simulink model "hpt_topology1_tutorial"  (R2025a)
settings: Solver=FixedStepDiscrete  StartTime=0.0  StopTime=0.25  FixedStep=Ts_power  RelTol=1e-3
model workspace (MAT data in the model file):
  Cdc_nom = 0.0022
  I_energy_max = 220
  K_vdc = 0.0018
  K_vreg = -0.03
  L_w5_open = 0
  Lg_grid = 0.262592258879
  P_load = 400000
  Q_load_cap = 0
  Q_load_ind = 0
  R_w4_open = 1000000000
  R_w5_open = 1000000000
  Rg_grid = 11.7851130198
  SCR_grid = 3
  S_base = 400000
  S_energy = 120000
  S_main = 400000
  S_series = 30000
  Ts_power = 2e-05
  Vaux_LL = 400
  Vdc_chopper_on = 850
  Vdc_neg_ref = 0
  Vdc_nom = 800
  Vdc_ref = 875
  Vgrid_LL = 11000
  Vinj_w5_phase_peak = 326.598632371
  Vload_LL = 400
  Vlv_LL = 400
  Vlv_ref_phase = 207
  Vmv_LL = 10000
  Vw5_reg = 400
  Vw6_series = 100
  f_grid = 50
  hpt_energy_auto = 1
  hpt_pwm_fs = 2000
  hpt_vreg_auto = 1
  m_energy_limit = 1.5
  m_energy_manual = 0
  m_reg_limit = 0.6
  m_reg_manual = 0
  omega_grid = 314.159265359
  vdc_lpf_alpha = 0.004
  vreg_lpf_alpha = 0.004
libraries: simulink x9, spsLinearTransformerLib x6, spsUniversalBridgeLib x4, spsGroundLib x3, spsThreePhaseVIMeasurementLib x2, spsSeriesRLCBranchLib x1, spsVoltageMeasurementLib x1, spsControlledCurrentSourceLib x1, spsThreePhaseSourceLib x1, spsThreePhaseSeriesRLCLoadLib x1, spsThreePhaseSeriesRLCBranchLib x1, sps_lib x1
settings Model: Creator=m1391  LastModifiedBy=m1391

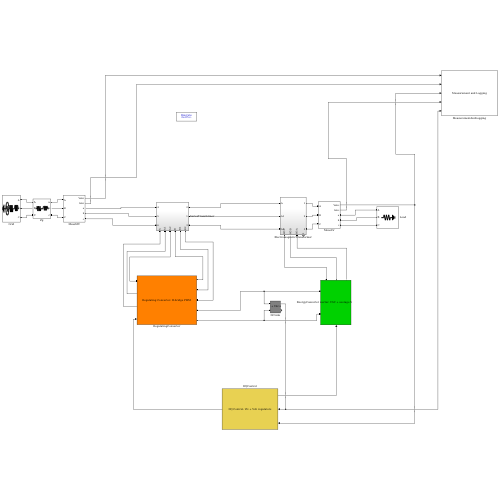
[thumbnail: Simulink's stored preview of the top-level diagram]
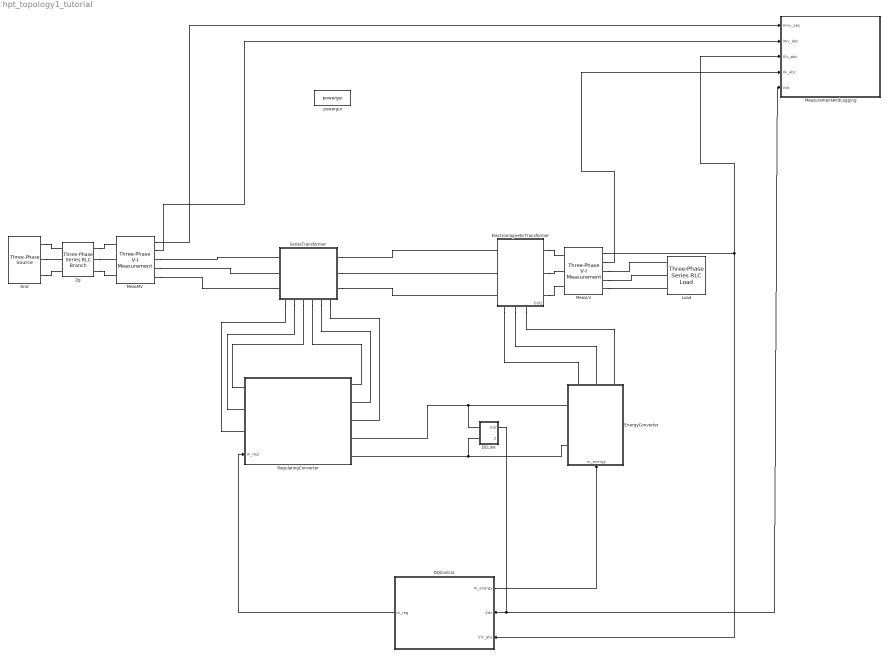
== system hpt_topology1_tutorial ==
  DCLink : Subsystem
      mask Display: disp('DC Link: Cdc + Vdc measurement');
  DQControl : Subsystem
      settings: PortSchema="{\"entries\":[{\"content\":{\"sides\":[{\"content\":{\"connectorIds\":[\"In1\",\"In2\",\"Out2\"]},\"type\":\"ConnectorPlacement.EquallySpacedRectSide\",\"uuid\":\"3cf5f39b-346d-4845-a4cb-051bfc2b4b05\"},{\"content\":{\"connectorIds\":[\"Out1\"],\"side\":\"RIGHT\"},\"type\":\"ConnectorPlacement.EquallySpacedRectSide\",\"uuid\":\"ecd50919-0b1c-4c05-b48e-325f2eadaf48\"},{\"content\":{\"side\":\"TOP\"},\"type\":\"ConnectorPlacement.EquallySpacedRectSide\",\"uuid\":\"d29a4cd4-7c66-4d73-bb68-e387a593270b\"}]},\"type\":\"ConnectorPlacement.EquallySpacedConnector\",\"uuid\":\"966f23e7-eea6-45dc-87ce-60332307e870\"}],\"packageUris\":[\"http://schema.mathworks.com/mf0/Connector/R2020b\"],\"version\":\"1.0\"}"
      mask Display: disp('DQ Control: Vlv + Vdc regulators');
  ElectromagneticTransformer : Subsystem
      settings: PortSchema="{\"entries\":[{\"content\":{\"sides\":[{\"content\":{\"connectorIds\":[\"LConn1\",\"LConn2\",\"LConn3\"]},\"type\":\"ConnectorPlacement.EquallySpacedRectSide\",\"uuid\":\"a1b13bb1-2dce-4e6a-9079-2e847976adb7\"},{\"content\":{\"connectorIds\":[\"RConn1\",\"RConn2\",\"RConn3\"],\"side\":\"RIGHT\"},\"type\":\"ConnectorPlacement.EquallySpacedRectSide\",\"uuid\":\"d74f82ee-ef21-4deb-91b0-5013dd9f5252\"},{\"content\":{\"side\":\"TOP\"},\"type\":\"ConnectorPlacement.EquallySpacedRectSide\",\"uuid\":\"c8027a0e-7a63-44e2-8b0b-a3b1c9bc6e6e\"},{\"content\":{\"connectorIds\":[\"RConn4\",\"RConn5\",\"RConn6\",\"Out1\"],\"side\":\"BOTTOM\"},\"type\":\"ConnectorPlacement.EquallySpacedRectSide\",\"uuid\":\"67c2655b-5962-44e1-8ca2-30aff8808cec\"}]},\"type\":\"ConnectorPlacement.EquallySpacedConnector\",\"uuid\":\"b1661991-e7ef-4d20-9f05-05442b8b5b75\"}],\"packageUris\":[\"http://schema.mathworks.com/mf0/Connector/R2020b\"],\"version\":\"1.0\"}"
  EnergyConverter : Subsystem
      settings: PortSchema="{\"entries\":[{\"content\":{\"sides\":[{\"content\":{\"connectorIds\":[\"LConn1\",\"LConn2\",\"LConn3\"]},\"type\":\"ConnectorPlacement.EquallySpacedRectSide\",\"uuid\":\"97f6e42d-fadd-43ac-9276-7e2aa194abfa\"},{\"content\":{\"connectorIds\":[\"In1\"],\"side\":\"RIGHT\"},\"type\":\"ConnectorPlacement.EquallySpacedRectSide\",\"uuid\":\"de6186ba-5c28-4c9b-a5f0-012c988ed5c8\"},{\"content\":{\"side\":\"TOP\"},\"type\":\"ConnectorPlacement.EquallySpacedRectSide\",\"uuid\":\"44ac97f7-235b-401f-a006-13d9f71848c4\"},{\"content\":{\"connectorIds\":[\"RConn1\",\"RConn2\"],\"side\":\"BOTTOM\"},\"type\":\"ConnectorPlacement.EquallySpacedRectSide\",\"uuid\":\"a31777c4-3c51-48d3-9206-785db4191288\"}]},\"type\":\"ConnectorPlacement.EquallySpacedConnector\",\"uuid\":\"4528e4fd-5330-48b9-923f-21a37255ca08\"}],\"packageUris\":[\"http://schema.mathworks.com/mf0/Connector/R2020b\"],\"version\":\"1.0\"}"
      mask Display: disp('Energy Converter: VSC + average Vdc support');
  Grid : spsThreePhaseSourceLib/Three-Phase Source  InternalConnection=Yg  VoltagePhases=off  Voltage=Vgrid_LL  PhaseAngle=0  Voltage_phases=[25e3 25e3 25e3]/sqrt(3)  PhaseAngles_phases=[0 -120 +120]  Frequency=f_grid  NonIdealSource=on  SpecifyImpedance=off  Resistance=1e-3  Inductance=1e-5  ShortCircuitLevel=100e6  BaseVoltage=25e3  XRratio=7  BusType=swing  Pref=10e3  Qref=0  Prefabc=[10e3, 10e3, 10e3]  Qrefabc=[0, 0, 0]  Qmin=-inf  Qmax=inf
  Load : spsThreePhaseSeriesRLCLoadLib/Three-Phase Series RLC Load  LConnTagsString=A|B|C  Configuration=Y (grounded)  NominalVoltage=Vload_LL  Vabc=[1e3 1e3 1e3]  Vabcp=[1e3 1e3 1e3]  NominalFrequency=f_grid  UnbalancedPower=off  ActivePower=P_load  InductivePower=Q_load_ind  CapacitivePower=Q_load_cap  Pabc=[10e3 9e3 11e3]  QLabc=[100 90 110]  QCabc=[100 90 110]  Pabcp=[10e3 9e3 11e3]  QLabcp=[100 90 110]  QCabcp=[100 90 110]  Measurements=None  LoadType=constant Z
  MeasLV : spsThreePhaseVIMeasurementLib/Three-Phase V-I Measurement  VoltageMeasurement=phase-to-ground  SetLabelV=off  LabelV=Vabc  Vpu=off  VpuLL=off  CurrentMeasurement=yes  SetLabelI=off  LabelI=Iabc  Ipu=off  Pbase=100e6  Vbase=500e3  OutputType=Complex  PhasorSimulation=off  PSBequivalent=0
  MeasMV : spsThreePhaseVIMeasurementLib/Three-Phase V-I Measurement  VoltageMeasurement=phase-to-ground  SetLabelV=off  LabelV=Vabc  Vpu=off  VpuLL=off  CurrentMeasurement=yes  SetLabelI=off  LabelI=Iabc  Ipu=off  Pbase=100e6  Vbase=500e3  OutputType=Complex  PhasorSimulation=off  PSBequivalent=0
  MeasurementAndLogging : Subsystem
      mask Display: disp('Measurement and Logging');
  RegulatingConverter : Subsystem
      settings: PortSchema="{\"entries\":[{\"content\":{\"sides\":[{\"content\":{\"connectorIds\":[\"LConn1\",\"LConn2\",\"LConn3\",\"In1\"]},\"type\":\"ConnectorPlacement.EquallySpacedRectSide\",\"uuid\":\"97f6e42d-fadd-43ac-9276-7e2aa194abfa\"},{\"content\":{\"connectorIds\":[\"RConn1\",\"RConn2\",\"RConn3\",\"RConn4\",\"RConn5\"],\"side\":\"RIGHT\"},\"type\":\"ConnectorPlacement.EquallySpacedRectSide\",\"uuid\":\"de6186ba-5c28-4c9b-a5f0-012c988ed5c8\"},{\"content\":{\"side\":\"TOP\"},\"type\":\"ConnectorPlacement.EquallySpacedRectSide\",\"uuid\":\"44ac97f7-235b-401f-a006-13d9f71848c4\"}]},\"type\":\"ConnectorPlacement.EquallySpacedConnector\",\"uuid\":\"4528e4fd-5330-48b9-923f-21a37255ca08\"}],\"packageUris\":[\"http://schema.mathworks.com/mf0/Connector/R2020b\"],\"version\":\"1.0\"}"
      mask Display: disp('Regulating Converter: H-bridge PWM');
  SeriesTransformer : Subsystem
      settings: PortSchema="{\"entries\":[{\"content\":{\"sides\":[{\"content\":{\"connectorIds\":[\"LConn1\",\"LConn2\",\"LConn3\",\"LConn4\",\"LConn5\",\"LConn6\"]},\"type\":\"ConnectorPlacement.EquallySpacedRectSide\",\"uuid\":\"20d82d84-5695-4c20-a185-fbc9bc49a76c\"},{\"content\":{\"side\":\"RIGHT\"},\"type\":\"ConnectorPlacement.EquallySpacedRectSide\",\"uuid\":\"33b448d8-8c06-4227-825b-ecd8e4ec0e04\"},{\"content\":{\"connectorIds\":[\"LConn7\",\"LConn8\",\"LConn9\"],\"side\":\"TOP\"},\"type\":\"ConnectorPlacement.EquallySpacedRectSide\",\"uuid\":\"ab355161-f222-40c3-9b59-8845a3e0aeb1\"},{\"content\":{\"connectorIds\":[\"RConn1\",\"RConn2\",\"RConn3\"],\"side\":\"BOTTOM\"},\"type\":\"ConnectorPlacement.EquallySpacedRectSide\",\"uuid\":\"91de8b9a-4f62-4b4f-95bb-28c45509e8d0\"}]},\"type\":\"ConnectorPlacement.EquallySpacedConnector\",\"uuid\":\"d2e8fda0-d220-450b-a404-ca6f656a2c35\"}],\"packageUris\":[\"http://schema.mathworks.com/mf0/Connector/R2020b\"],\"version\":\"1.0\"}"
  Zg : spsThreePhaseSeriesRLCBranchLib/Three-Phase Series RLC Branch  LConnTagsString=A|B|C  RConnTagsString=A|B|C  BranchType=RL  Resistance=Rg_grid  Inductance=Lg_grid  Capacitance=1e-6  Measurements=None
  powergui : sps_lib/powergui  Priority=1  SimulationMode=Discrete  SampleTime=Ts_power  frequency=60  Iterations=50  frequencyindice=50  Pbase=100e6  ErrMax=1e-4  UnitsV=kV  UnitsW=MW  buscounter=0  FunctionMessages=off  echomessages=off  EnableUseOfTLC=off  CurrentSourceSwitches=off  DisableSnubberDevices=off  DisableRonSwitches=off  DisableVfSwitches=off  DisplayEquations=off  AutomaticDiscreteSolvers=off  SolverType=Tustin/Backward Euler (TBE)  Interpol=off  ExternalGateDelay=off  methode=off  Ts=100  x0status=blocks  SPID=on  SwTol=0  HookPort=off  NonlinearTolerance=1e-4  nMaxIteration=100  ContinueOnMaxIteration=off  RestoreLinks=warning  ResistiveCurrentMeasurement=off  Frange=[0:2:500]  Ylog=off  Xlog=on  ShowGrid=off  save=off  variable=ZData  structure=0  ZoomFFT=off  StartTime=0.0  cycles=1  DisplayStyle=1  fundamental=60  FreqAxis=off  MaxFrequency=1000  frequencyindicesteady=1  RmsSteady=1  display=off
  wires:
  DCLink/1(Vdc) -> MeasurementAndLogging/5(Vdc), DQControl/2(Vdc)
  MeasMV/1 -> MeasurementAndLogging/1(Vmv_abc)
  MeasMV/2 -> MeasurementAndLogging/2(Imv_abc)
  MeasLV/1 -> MeasurementAndLogging/3(Vlv_abc), DQControl/1(Vlv_abc)
  MeasLV/2 -> MeasurementAndLogging/4(Ilv_abc)
  DQControl/1(m_reg) -> RegulatingConverter/1(m_reg)
  DQControl/2(m_energy) -> EnergyConverter/1(m_energy)
  connections:
  Grid/RConn1 -- Zg/LConn1
  Zg/RConn1 -- MeasMV/LConn1
  Grid/RConn2 -- Zg/LConn2
  Zg/RConn2 -- MeasMV/LConn2
  Grid/RConn3 -- Zg/LConn3
  Zg/RConn3 -- MeasMV/LConn3
  MeasLV/RConn1 -- Load/LConn1
  MeasLV/RConn2 -- Load/LConn2
  MeasLV/RConn3 -- Load/LConn3
  SeriesTransformer/LConn1 -- RegulatingConverter/LConn3
  SeriesTransformer/LConn4 -- RegulatingConverter/RConn1
  SeriesTransformer/LConn2 -- RegulatingConverter/LConn2
  SeriesTransformer/LConn5 -- RegulatingConverter/RConn2
  SeriesTransformer/LConn3 -- RegulatingConverter/LConn1
  SeriesTransformer/LConn6 -- RegulatingConverter/RConn3
  SeriesTransformer/RConn3 -- ElectromagneticTransformer/LConn1
  SeriesTransformer/RConn2 -- ElectromagneticTransformer/LConn2
  SeriesTransformer/RConn1 -- ElectromagneticTransformer/LConn3
  MeasMV/RConn1 -- SeriesTransformer/LConn9
  MeasMV/RConn2 -- SeriesTransformer/LConn8
  MeasMV/RConn3 -- SeriesTransformer/LConn7
  DCLink/LConn1 -- RegulatingConverter/RConn4 -- EnergyConverter/RConn1
  DCLink/LConn2 -- RegulatingConverter/RConn5 -- EnergyConverter/RConn2
  ElectromagneticTransformer/RConn1 -- MeasLV/LConn1
  ElectromagneticTransformer/RConn6 -- EnergyConverter/LConn1
  ElectromagneticTransformer/RConn2 -- MeasLV/LConn2
  ElectromagneticTransformer/RConn5 -- EnergyConverter/LConn2
  ElectromagneticTransformer/RConn3 -- MeasLV/LConn3
  ElectromagneticTransformer/RConn4 -- EnergyConverter/LConn3

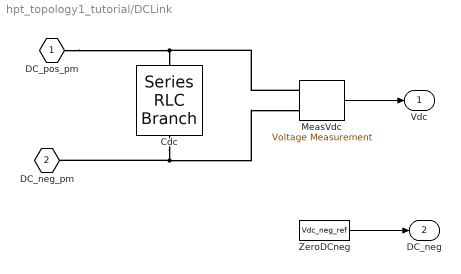
== system hpt_topology1_tutorial/DCLink ==
  Cdc : spsSeriesRLCBranchLib/Series RLC Branch  LConnTagsString=__new0  RConnTagsString=__new0  BranchType=C  Resistance=1  Inductance=1e-3  SetiL0=off  InitialCurrent=0  Capacitance=Cdc_nom  Setx0=off  InitialVoltage=Vdc_nom  Measurements=None
  MeasVdc : spsVoltageMeasurementLib/Voltage Measurement  PhasorSimulation=off  OutputType=Complex  PSBequivalent=0
  ZeroDCneg : Constant  Value=Vdc_neg_ref
  DC_pos_pm : PMIOPort  Side=Left
  DC_neg_pm : PMIOPort  Port=2  Side=Left
  Vdc : Outport
  DC_neg : Outport  Port=2
  wires:
  MeasVdc/1 -> Vdc/1
  ZeroDCneg/1 -> DC_neg/1
  connections:
  DC_pos_pm/RConn1 -- MeasVdc/LConn1 -- Cdc/LConn1
  DC_neg_pm/RConn1 -- MeasVdc/LConn2 -- Cdc/RConn1

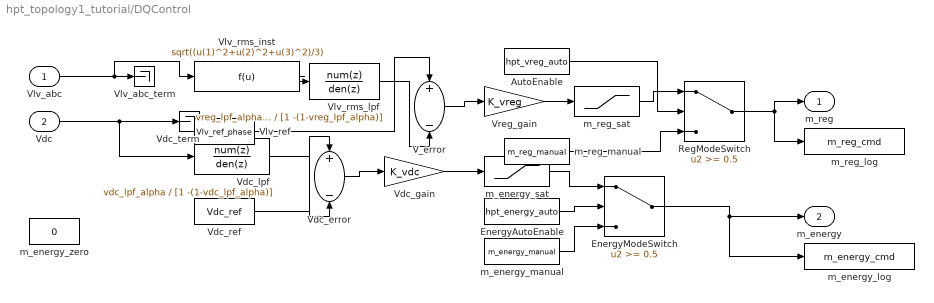
== system hpt_topology1_tutorial/DQControl ==
  Vlv_abc : Inport
  Vdc : Inport  Port=2
  AutoEnable : Constant  Value=hpt_vreg_auto
  EnergyAutoEnable : Constant  Value=hpt_energy_auto
  EnergyModeSwitch : Switch  Threshold=0.5  SaturateOnIntegerOverflow=off  InputSameDT=off
  RegModeSwitch : Switch  Threshold=0.5  SaturateOnIntegerOverflow=off  InputSameDT=off
  V_error : Sum  Inputs=+-
  Vdc_error : Sum  Inputs=+-
  Vdc_gain : Gain  Gain=K_vdc
  Vdc_lpf : DiscreteTransferFcn  Numerator=vdc_lpf_alpha  Denominator=[1 -(1-vdc_lpf_alpha)]  SampleTime=Ts_power
  Vdc_ref : Constant  Value=Vdc_ref
  Vdc_term : Terminator
  Vlv_abc_term : Terminator
  Vlv_ref : Constant  Value=Vlv_ref_phase
  Vlv_rms_inst : Fcn  Expr=sqrt((u(1)^2+u(2)^2+u(3)^2)/3)
  Vlv_rms_lpf : DiscreteTransferFcn  Numerator=vreg_lpf_alpha  Denominator=[1 -(1-vreg_lpf_alpha)]  SampleTime=Ts_power
  Vreg_gain : Gain  Gain=K_vreg
  m_energy_log : ToWorkspace  VariableName=m_energy_cmd  SampleTime=Ts_power
  m_energy_manual : Constant  Value=m_energy_manual
  m_energy_sat : Saturate  UpperLimit=m_energy_limit  LowerLimit=-m_energy_limit
  m_energy_zero : Constant  Value=0
  m_reg_log : ToWorkspace  VariableName=m_reg_cmd  SampleTime=Ts_power
  m_reg_manual : Constant  Value=m_reg_manual
  m_reg_sat : Saturate  UpperLimit=m_reg_limit  LowerLimit=-m_reg_limit
  m_reg : Outport
  m_energy : Outport  Port=2
  wires:
  Vlv_abc/1 -> Vlv_abc_term/1, Vlv_rms_inst/1
  Vdc/1 -> Vdc_term/1, Vdc_lpf/1
  Vlv_ref/1 -> V_error/1
  V_error/1 -> Vreg_gain/1
  Vreg_gain/1 -> m_reg_sat/1
  m_reg_sat/1 -> RegModeSwitch/1
  AutoEnable/1 -> RegModeSwitch/2
  m_reg_manual/1 -> RegModeSwitch/3
  RegModeSwitch/1 -> m_reg/1, m_reg_log/1
  Vlv_rms_inst/1 -> Vlv_rms_lpf/1
  Vlv_rms_lpf/1 -> V_error/2
  Vdc_ref/1 -> Vdc_error/1
  Vdc_lpf/1 -> Vdc_error/2
  Vdc_error/1 -> Vdc_gain/1
  Vdc_gain/1 -> m_energy_sat/1
  m_energy_sat/1 -> EnergyModeSwitch/1
  EnergyAutoEnable/1 -> EnergyModeSwitch/2
  m_energy_manual/1 -> EnergyModeSwitch/3
  EnergyModeSwitch/1 -> m_energy/1, m_energy_log/1

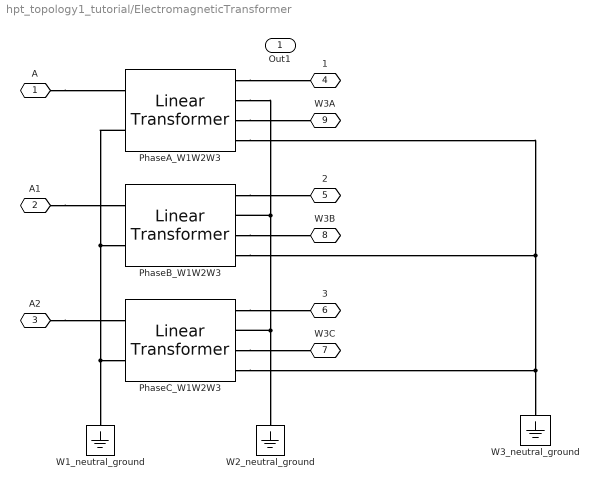
== system hpt_topology1_tutorial/ElectromagneticTransformer ==
  PhaseA_W1W2W3 : spsLinearTransformerLib/Linear Transformer  UNITS=pu  NominalPower=[S_main/3,f_grid]  winding1=[Vmv_LL/sqrt(3),0.005,0.025]  winding2=[Vlv_LL/sqrt(3),0.005,0.025]  ThreeWindings=on  winding3=[Vaux_LL/sqrt(3),0.005,0.02]  RmLm=[ 500 500 ]  Measurements=None  DataType=off
  PhaseB_W1W2W3 : spsLinearTransformerLib/Linear Transformer  UNITS=pu  NominalPower=[S_main/3,f_grid]  winding1=[Vmv_LL/sqrt(3),0.005,0.025]  winding2=[Vlv_LL/sqrt(3),0.005,0.025]  ThreeWindings=on  winding3=[Vaux_LL/sqrt(3),0.005,0.02]  RmLm=[ 500 500 ]  Measurements=None  DataType=off
  PhaseC_W1W2W3 : spsLinearTransformerLib/Linear Transformer  UNITS=pu  NominalPower=[S_main/3,f_grid]  winding1=[Vmv_LL/sqrt(3),0.005,0.025]  winding2=[Vlv_LL/sqrt(3),0.005,0.025]  ThreeWindings=on  winding3=[Vaux_LL/sqrt(3),0.005,0.02]  RmLm=[ 500 500 ]  Measurements=None  DataType=off
  W1_neutral_ground : spsGroundLib/Ground  LConnTagsString=a
  W2_neutral_ground : spsGroundLib/Ground  LConnTagsString=a
  W3_neutral_ground : spsGroundLib/Ground  LConnTagsString=a
  A : PMIOPort  Side=Left
  A1 : PMIOPort  Port=2  Side=Left
  A2 : PMIOPort  Port=3  Side=Left
  1 : PMIOPort  Port=4  Side=Right
  2 : PMIOPort  Port=5  Side=Right
  3 : PMIOPort  Port=6  Side=Right
  W3C : PMIOPort  Port=7  Side=Right
  W3B : PMIOPort  Port=8  Side=Right
  W3A : PMIOPort  Port=9  Side=Right
  Out1 : Outport
  connections:
  PhaseA_W1W2W3/RConn1 -- 1/RConn1
  PhaseC_W1W2W3/RConn1 -- 3/RConn1
  PhaseA_W1W2W3/RConn2 -- W2_neutral_ground/LConn1 -- PhaseC_W1W2W3/RConn2 -- PhaseB_W1W2W3/RConn2
  PhaseA_W1W2W3/LConn2 -- PhaseB_W1W2W3/LConn2 -- PhaseC_W1W2W3/LConn2 -- W1_neutral_ground/LConn1
  A/RConn1 -- PhaseA_W1W2W3/LConn1
  A1/RConn1 -- PhaseB_W1W2W3/LConn1
  PhaseB_W1W2W3/RConn1 -- 2/RConn1
  A2/RConn1 -- PhaseC_W1W2W3/LConn1
  PhaseA_W1W2W3/RConn3 -- W3A/RConn1
  PhaseA_W1W2W3/RConn4 -- PhaseB_W1W2W3/RConn4 -- PhaseC_W1W2W3/RConn4 -- W3_neutral_ground/LConn1
  PhaseB_W1W2W3/RConn3 -- W3B/RConn1
  PhaseC_W1W2W3/RConn3 -- W3C/RConn1

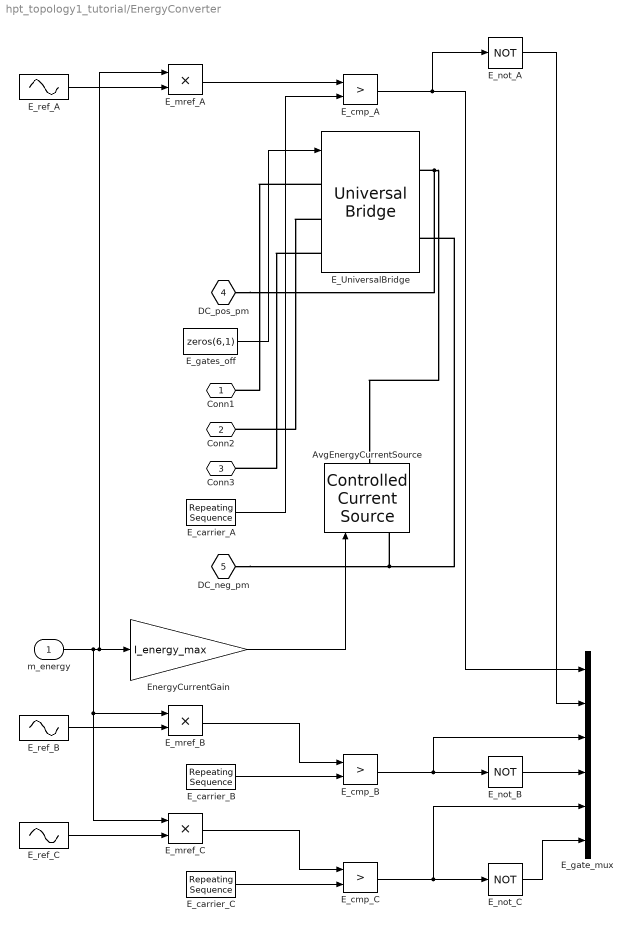
== system hpt_topology1_tutorial/EnergyConverter ==
  m_energy : Inport
  AvgEnergyCurrentSource : spsControlledCurrentSourceLib/Controlled Current Source  Initialize=on  Source_Type=AC  Amplitude=0  Phase=0  Frequency=0  Measurements=None
  E_UniversalBridge : spsUniversalBridgeLib/Universal Bridge  Arms=3  SnubberResistance=1e5  SnubberCapacitance=1e-9  Device=IGBT / Diodes  Ron=1e-3  Lon=0  ForwardVoltages="[  0  0  ]"  ForwardVoltage=0  GTOparameters=[ 10e-6 , 20e-6 ]  IGBTparameters=[ 1e-6 , 2e-6 ]  Measurements=None  Measurements_2=None  converterType=Rectifier
  E_carrier_A : simulink/Sources/Repeating Sequence  rep_seq_t=[0 0.5/hpt_pwm_fs 1/hpt_pwm_fs]  rep_seq_y=[-1 1 -1]
  E_carrier_B : simulink/Sources/Repeating Sequence  rep_seq_t=[0 0.5/hpt_pwm_fs 1/hpt_pwm_fs]  rep_seq_y=[-1 1 -1]
  E_carrier_C : simulink/Sources/Repeating Sequence  rep_seq_t=[0 0.5/hpt_pwm_fs 1/hpt_pwm_fs]  rep_seq_y=[-1 1 -1]
  E_cmp_A : RelationalOperator  Operator=>  OutDataTypeStr=boolean  RndMeth=Simplest  InputSameDT=off
  E_cmp_B : RelationalOperator  Operator=>  OutDataTypeStr=boolean  RndMeth=Simplest  InputSameDT=off
  E_cmp_C : RelationalOperator  Operator=>  OutDataTypeStr=boolean  RndMeth=Simplest  InputSameDT=off
  E_gate_mux : Mux  Inputs=6
  E_gates_off : Constant  Value=zeros(6,1)
  E_mref_A : Product  Inputs=**
  E_mref_B : Product  Inputs=**
  E_mref_C : Product  Inputs=**
  E_not_A : Logic  Operator=NOT  AllPortsSameDT=off  OutDataTypeStr=boolean
  E_not_B : Logic  Operator=NOT  AllPortsSameDT=off  OutDataTypeStr=boolean
  E_not_C : Logic  Operator=NOT  AllPortsSameDT=off  OutDataTypeStr=boolean
  E_ref_A : Sin  Frequency=2*pi*50  SampleTime=0
  E_ref_B : Sin  Frequency=2*pi*50  Phase=-2*pi/3  SampleTime=0
  E_ref_C : Sin  Frequency=2*pi*50  Phase=2*pi/3  SampleTime=0
  EnergyCurrentGain : Gain  Gain=I_energy_max
  Conn1 : PMIOPort  Side=Left
  Conn2 : PMIOPort  Port=2  Side=Left
  Conn3 : PMIOPort  Port=3  Side=Left
  DC_pos_pm : PMIOPort  Port=4  Side=Right
  DC_neg_pm : PMIOPort  Port=5  Side=Right
  wires:
  E_ref_A/1 -> E_mref_A/2
  E_not_B/1 -> E_gate_mux/4
  E_ref_C/1 -> E_mref_C/2
  m_energy/1 -> E_mref_B/1, E_mref_C/1, E_mref_A/1, EnergyCurrentGain/1
  E_gates_off/1 -> E_UniversalBridge/1
  E_ref_B/1 -> E_mref_B/2
  E_mref_A/1 -> E_cmp_A/1
  E_carrier_A/1 -> E_cmp_A/2
  EnergyCurrentGain/1 -> AvgEnergyCurrentSource/1
  E_mref_B/1 -> E_cmp_B/1
  E_carrier_B/1 -> E_cmp_B/2
  E_mref_C/1 -> E_cmp_C/1
  E_carrier_C/1 -> E_cmp_C/2
  E_cmp_A/1 -> E_gate_mux/1, E_not_A/1
  E_not_A/1 -> E_gate_mux/2
  E_cmp_B/1 -> E_gate_mux/3, E_not_B/1
  E_cmp_C/1 -> E_gate_mux/5, E_not_C/1
  E_not_C/1 -> E_gate_mux/6
  connections:
  DC_pos_pm/RConn1 -- AvgEnergyCurrentSource/RConn1 -- E_UniversalBridge/RConn1
  DC_neg_pm/RConn1 -- AvgEnergyCurrentSource/LConn1 -- E_UniversalBridge/RConn2
  E_UniversalBridge/LConn3 -- Conn3/RConn1
  E_UniversalBridge/LConn2 -- Conn2/RConn1
  E_UniversalBridge/LConn1 -- Conn1/RConn1

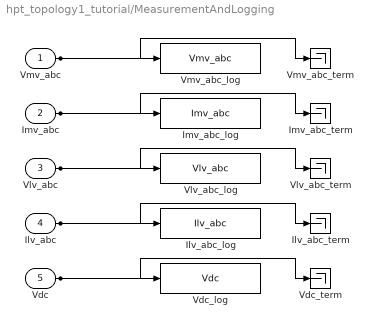
== system hpt_topology1_tutorial/MeasurementAndLogging ==
  Vmv_abc : Inport
  Imv_abc : Inport  Port=2
  Vlv_abc : Inport  Port=3
  Ilv_abc : Inport  Port=4
  Vdc : Inport  Port=5
  Ilv_abc_log : ToWorkspace  VariableName=Ilv_abc  SampleTime=Ts_power
  Ilv_abc_term : Terminator
  Imv_abc_log : ToWorkspace  VariableName=Imv_abc  SampleTime=Ts_power
  Imv_abc_term : Terminator
  Vdc_log : ToWorkspace  VariableName=Vdc  SampleTime=Ts_power
  Vdc_term : Terminator
  Vlv_abc_log : ToWorkspace  VariableName=Vlv_abc  SampleTime=Ts_power
  Vlv_abc_term : Terminator
  Vmv_abc_log : ToWorkspace  VariableName=Vmv_abc  SampleTime=Ts_power
  Vmv_abc_term : Terminator
  wires:
  Vmv_abc/1 -> Vmv_abc_log/1, Vmv_abc_term/1
  Imv_abc/1 -> Imv_abc_log/1, Imv_abc_term/1
  Vlv_abc/1 -> Vlv_abc_log/1, Vlv_abc_term/1
  Ilv_abc/1 -> Ilv_abc_log/1, Ilv_abc_term/1
  Vdc/1 -> Vdc_log/1, Vdc_term/1

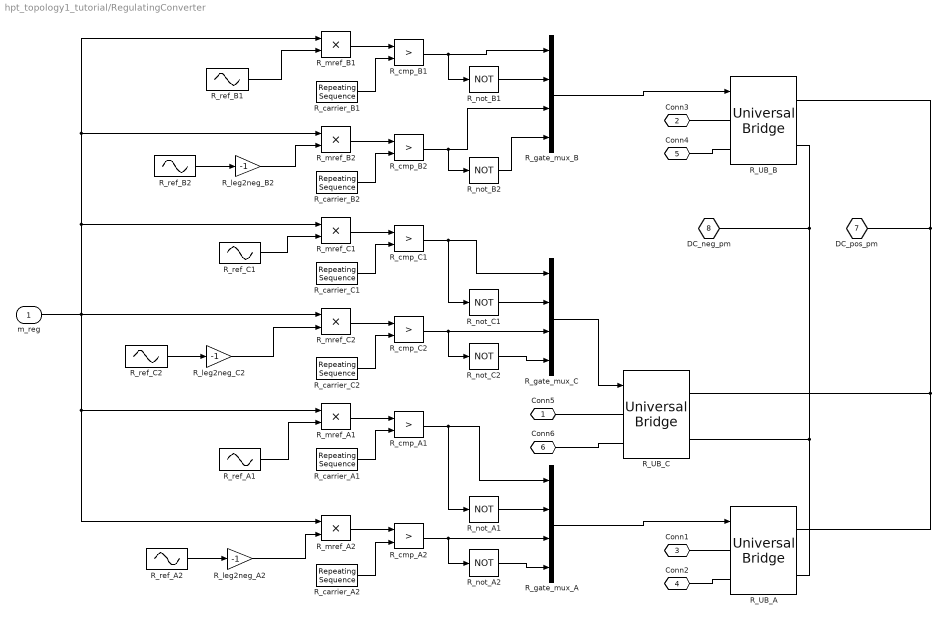
== system hpt_topology1_tutorial/RegulatingConverter ==
  m_reg : Inport
  R_UB_A : spsUniversalBridgeLib/Universal Bridge  Arms=2  SnubberResistance=1e5  SnubberCapacitance=1e-9  Device=IGBT / Diodes  Ron=1e-3  Lon=0  ForwardVoltages="[  0  0  ]"  ForwardVoltage=0  GTOparameters=[ 10e-6 , 20e-6 ]  IGBTparameters=[ 1e-6 , 2e-6 ]  Measurements=None  Measurements_2=None  converterType=Rectifier
  R_UB_B : spsUniversalBridgeLib/Universal Bridge  Arms=2  SnubberResistance=1e5  SnubberCapacitance=1e-9  Device=IGBT / Diodes  Ron=1e-3  Lon=0  ForwardVoltages="[  0  0  ]"  ForwardVoltage=0  GTOparameters=[ 10e-6 , 20e-6 ]  IGBTparameters=[ 1e-6 , 2e-6 ]  Measurements=None  Measurements_2=None  converterType=Rectifier
  R_UB_C : spsUniversalBridgeLib/Universal Bridge  Arms=2  SnubberResistance=1e5  SnubberCapacitance=1e-9  Device=IGBT / Diodes  Ron=1e-3  Lon=0  ForwardVoltages="[  0  0  ]"  ForwardVoltage=0  GTOparameters=[ 10e-6 , 20e-6 ]  IGBTparameters=[ 1e-6 , 2e-6 ]  Measurements=None  Measurements_2=None  converterType=Rectifier
  R_carrier_A1 : simulink/Sources/Repeating Sequence  rep_seq_t=[0 0.5/hpt_pwm_fs 1/hpt_pwm_fs]  rep_seq_y=[-1 1 -1]
  R_carrier_A2 : simulink/Sources/Repeating Sequence  rep_seq_t=[0 0.5/hpt_pwm_fs 1/hpt_pwm_fs]  rep_seq_y=[-1 1 -1]
  R_carrier_B1 : simulink/Sources/Repeating Sequence  rep_seq_t=[0 0.5/hpt_pwm_fs 1/hpt_pwm_fs]  rep_seq_y=[-1 1 -1]
  R_carrier_B2 : simulink/Sources/Repeating Sequence  rep_seq_t=[0 0.5/hpt_pwm_fs 1/hpt_pwm_fs]  rep_seq_y=[-1 1 -1]
  R_carrier_C1 : simulink/Sources/Repeating Sequence  rep_seq_t=[0 0.5/hpt_pwm_fs 1/hpt_pwm_fs]  rep_seq_y=[-1 1 -1]
  R_carrier_C2 : simulink/Sources/Repeating Sequence  rep_seq_t=[0 0.5/hpt_pwm_fs 1/hpt_pwm_fs]  rep_seq_y=[-1 1 -1]
  R_cmp_A1 : RelationalOperator  Operator=>  OutDataTypeStr=boolean  RndMeth=Simplest  InputSameDT=off
  R_cmp_A2 : RelationalOperator  Operator=>  OutDataTypeStr=boolean  RndMeth=Simplest  InputSameDT=off
  R_cmp_B1 : RelationalOperator  Operator=>  OutDataTypeStr=boolean  RndMeth=Simplest  InputSameDT=off
  R_cmp_B2 : RelationalOperator  Operator=>  OutDataTypeStr=boolean  RndMeth=Simplest  InputSameDT=off
  R_cmp_C1 : RelationalOperator  Operator=>  OutDataTypeStr=boolean  RndMeth=Simplest  InputSameDT=off
  R_cmp_C2 : RelationalOperator  Operator=>  OutDataTypeStr=boolean  RndMeth=Simplest  InputSameDT=off
  R_gate_mux_A : Mux
  R_gate_mux_B : Mux
  R_gate_mux_C : Mux
  R_leg2neg_A2 : Gain  Gain=-1
  R_leg2neg_B2 : Gain  Gain=-1
  R_leg2neg_C2 : Gain  Gain=-1
  R_mref_A1 : Product  Inputs=**
  R_mref_A2 : Product  Inputs=**
  R_mref_B1 : Product  Inputs=**
  R_mref_B2 : Product  Inputs=**
  R_mref_C1 : Product  Inputs=**
  R_mref_C2 : Product  Inputs=**
  R_not_A1 : Logic  Operator=NOT  AllPortsSameDT=off  OutDataTypeStr=boolean
  R_not_A2 : Logic  Operator=NOT  AllPortsSameDT=off  OutDataTypeStr=boolean
  R_not_B1 : Logic  Operator=NOT  AllPortsSameDT=off  OutDataTypeStr=boolean
  R_not_B2 : Logic  Operator=NOT  AllPortsSameDT=off  OutDataTypeStr=boolean
  R_not_C1 : Logic  Operator=NOT  AllPortsSameDT=off  OutDataTypeStr=boolean
  R_not_C2 : Logic  Operator=NOT  AllPortsSameDT=off  OutDataTypeStr=boolean
  R_ref_A1 : Sin  Frequency=2*pi*50  SampleTime=0
  R_ref_A2 : Sin  Frequency=2*pi*50  SampleTime=0
  R_ref_B1 : Sin  Frequency=2*pi*50  Phase=-2*pi/3  SampleTime=0
  R_ref_B2 : Sin  Frequency=2*pi*50  Phase=-2*pi/3  SampleTime=0
  R_ref_C1 : Sin  Frequency=2*pi*50  Phase=2*pi/3  SampleTime=0
  R_ref_C2 : Sin  Frequency=2*pi*50  Phase=2*pi/3  SampleTime=0
  Conn5 : PMIOPort  Side=Left
  Conn3 : PMIOPort  Port=2  Side=Left
  Conn1 : PMIOPort  Port=3  Side=Left
  Conn2 : PMIOPort  Port=4  Side=Right
  Conn4 : PMIOPort  Port=5  Side=Right
  Conn6 : PMIOPort  Port=6  Side=Right
  DC_pos_pm : PMIOPort  Port=7  Side=Right
  DC_neg_pm : PMIOPort  Port=8  Side=Right
  wires:
  R_not_B2/1 -> R_gate_mux_B/4
  R_leg2neg_C2/1 -> R_mref_C2/2
  R_carrier_B2/1 -> R_cmp_B2/2
  m_reg/1 -> R_mref_C2/1, R_mref_A1/1, R_mref_A2/1, R_mref_C1/1, R_mref_B2/1, R_mref_B1/1
  R_mref_C1/1 -> R_cmp_C1/1
  R_ref_B2/1 -> R_leg2neg_B2/1
  R_ref_C1/1 -> R_mref_C1/2
  R_not_C2/1 -> R_gate_mux_C/4
  R_ref_C2/1 -> R_leg2neg_C2/1
  R_ref_A2/1 -> R_leg2neg_A2/1
  R_ref_B1/1 -> R_mref_B1/2
  R_leg2neg_B2/1 -> R_mref_B2/2
  R_leg2neg_A2/1 -> R_mref_A2/2
  R_ref_A1/1 -> R_mref_A1/2
  R_mref_B1/1 -> R_cmp_B1/1
  R_carrier_B1/1 -> R_cmp_B1/2
  R_mref_B2/1 -> R_cmp_B2/1
  R_carrier_C1/1 -> R_cmp_C1/2
  R_mref_C2/1 -> R_cmp_C2/1
  R_carrier_C2/1 -> R_cmp_C2/2
  R_not_A2/1 -> R_gate_mux_A/4
  R_mref_A1/1 -> R_cmp_A1/1
  R_carrier_A1/1 -> R_cmp_A1/2
  R_mref_A2/1 -> R_cmp_A2/1
  R_carrier_A2/1 -> R_cmp_A2/2
  R_cmp_B1/1 -> R_gate_mux_B/1, R_not_B1/1
  R_cmp_B2/1 -> R_gate_mux_B/3, R_not_B2/1
  R_cmp_A1/1 -> R_gate_mux_A/1, R_not_A1/1
  R_cmp_C1/1 -> R_gate_mux_C/1, R_not_C1/1
  R_cmp_C2/1 -> R_gate_mux_C/3, R_not_C2/1
  R_cmp_A2/1 -> R_not_A2/1, R_gate_mux_A/3
  R_not_B1/1 -> R_gate_mux_B/2
  R_gate_mux_C/1 -> R_UB_C/1
  R_not_C1/1 -> R_gate_mux_C/2
  R_not_A1/1 -> R_gate_mux_A/2
  R_gate_mux_A/1 -> R_UB_A/1
  R_gate_mux_B/1 -> R_UB_B/1
  connections:
  Conn2/RConn1 -- R_UB_A/LConn2
  Conn5/RConn1 -- R_UB_C/LConn1
  Conn1/RConn1 -- R_UB_A/LConn1
  Conn3/RConn1 -- R_UB_B/LConn1
  DC_neg_pm/RConn1 -- R_UB_C/RConn2 -- R_UB_A/RConn2 -- R_UB_B/RConn2
  Conn6/RConn1 -- R_UB_C/LConn2
  Conn4/RConn1 -- R_UB_B/LConn2
  R_UB_C/RConn1 -- DC_pos_pm/RConn1 -- R_UB_B/RConn1 -- R_UB_A/RConn1

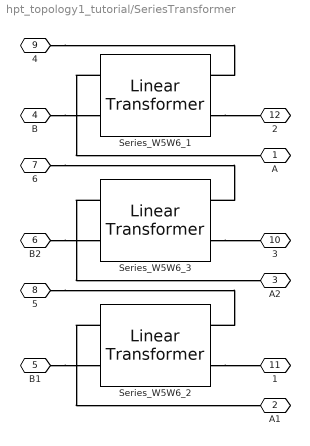
== system hpt_topology1_tutorial/SeriesTransformer ==
  Series_W5W6_1 : spsLinearTransformerLib/Linear Transformer  UNITS=pu  NominalPower=[S_series,f_grid]  winding1=[100,0.002,0.03]  winding2=[1600,0.002,0.03]  ThreeWindings=off  winding3=[ 315e3 0.002 0.08 ]  RmLm=[ 500 500 ]  Measurements=None  DataType=off
  Series_W5W6_2 : spsLinearTransformerLib/Linear Transformer  UNITS=pu  NominalPower=[S_series,f_grid]  winding1=[100,0.002,0.03]  winding2=[1600,0.002,0.03]  ThreeWindings=off  winding3=[ 315e3 0.002 0.08 ]  RmLm=[ 500 500 ]  Measurements=None  DataType=off
  Series_W5W6_3 : spsLinearTransformerLib/Linear Transformer  UNITS=pu  NominalPower=[S_series,f_grid]  winding1=[100,0.002,0.03]  winding2=[1600,0.002,0.03]  ThreeWindings=off  winding3=[ 315e3 0.002 0.08 ]  RmLm=[ 500 500 ]  Measurements=None  DataType=off
  A : PMIOPort  Side=Left
  A1 : PMIOPort  Port=2  Side=Left
  A2 : PMIOPort  Port=3  Side=Left
  B : PMIOPort  Port=4  Side=Left
  B1 : PMIOPort  Port=5  Side=Left
  B2 : PMIOPort  Port=6  Side=Left
  6 : PMIOPort  Port=7  Side=Left
  5 : PMIOPort  Port=8  Side=Left
  4 : PMIOPort  Port=9  Side=Left
  3 : PMIOPort  Port=10  Side=Right
  1 : PMIOPort  Port=11  Side=Right
  2 : PMIOPort  Port=12  Side=Right
  connections:
  B1/RConn1 -- Series_W5W6_2/LConn2
  Series_W5W6_1/LConn1 -- A/RConn1
  4/RConn1 -- Series_W5W6_1/RConn1
  B2/RConn1 -- Series_W5W6_3/LConn2
  Series_W5W6_1/RConn2 -- 2/RConn1
  B/RConn1 -- Series_W5W6_1/LConn2
  6/RConn1 -- Series_W5W6_3/RConn1
  5/RConn1 -- Series_W5W6_2/RConn1
  Series_W5W6_3/LConn1 -- A2/RConn1
  Series_W5W6_2/LConn1 -- A1/RConn1
  Series_W5W6_3/RConn2 -- 3/RConn1
  Series_W5W6_2/RConn2 -- 1/RConn1
